simulink model "llm_inferencing_control"  (R2025b)
settings: Solver=FixedStepDiscrete  StartTime=0.0  StopTime=300  FixedStep=perturbed.dt  RelTol=1e-3
undefined symbols (not defined in the file): perturbed
settings Model: Creator=hvasudevan  LastModifiedBy=hvasudevan

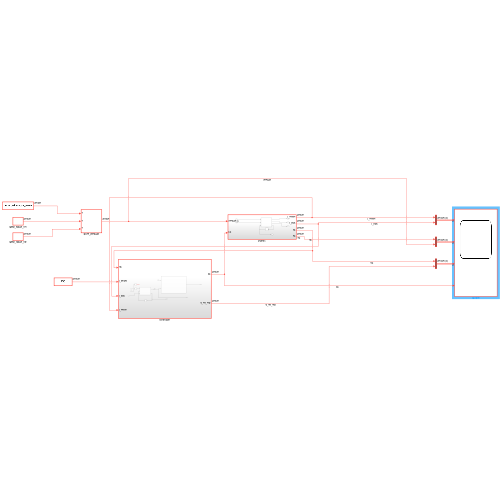
[thumbnail: Simulink's stored preview of the top-level diagram]
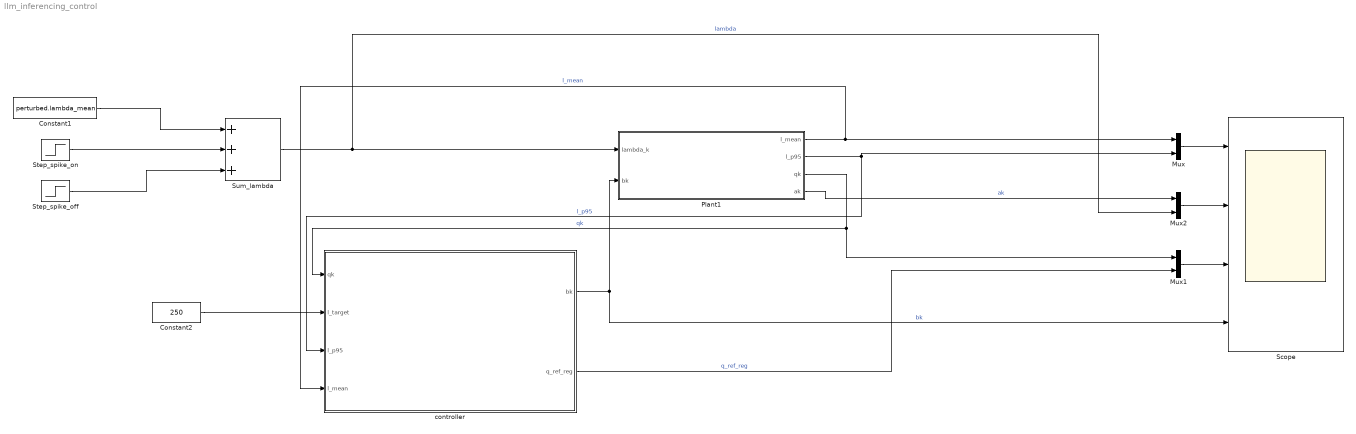
== system llm_inferencing_control ==
  Constant1 : Constant  Value=perturbed.lambda_mean  SampleTime=perturbed.dt
  Constant2 : Constant  Value=250  SampleTime=perturbed.dt
  Mux : Mux  Inputs=2
  Mux1 : Mux  Inputs=2
  Mux2 : Mux  Inputs=2
  Plant1 : Subsystem
  Scope : Scope  NumInputPorts=4
      settings: ActiveDisplayYMinimum=3.7725538298405183  ActiveDisplayYMaximum=466.04701553143548
  Step_spike_off : Step  Time=200  After=-perturbed.lambda_mean*1.5  SampleTime=perturbed.dt
  Step_spike_on : Step  Time=100  After=perturbed.lambda_mean*1.5  SampleTime=perturbed.dt
  Sum_lambda : Sum  Inputs=+++
  controller : Subsystem
  wires:
  Step_spike_off/1 -> Sum_lambda/3
  Plant1/3(qk) -> controller/1(qk), Mux1/1  "qk"
  Plant1/2(l_p95) -> Mux/2, controller/3(l_p95)  "l_p95"
  Plant1/1(l_mean) -> controller/4(l_mean), Mux/1  "l_mean"
  Step_spike_on/1 -> Sum_lambda/2
  Constant1/1 -> Sum_lambda/1
  Sum_lambda/1 -> Plant1/1(lambda_k), Mux2/2  "lambda"
  controller/1(bk) -> Scope/4, Plant1/2(bk)  "bk"
  Constant2/1 -> controller/2(l_target)
  Mux/1 -> Scope/1
  controller/2(q_ref_reg) -> Mux1/2  "q_ref_reg"
  Mux1/1 -> Scope/3
  Plant1/4(ak) -> Mux2/1  "ak"
  Mux2/1 -> Scope/2

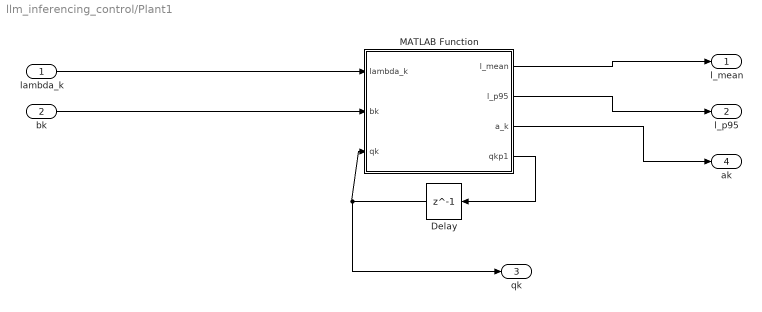
== system llm_inferencing_control/Plant1 ==
  lambda_k : Inport
  bk : Inport  Port=2
  Delay : Delay  DelayLength=1  InitialCondition=perturbed.q0  InputProcessing=Columns as channels (frame based)
  MATLAB Function : MATLAB Function  TreatAsAtomicUnit=on
  l_mean : Outport
  l_p95 : Outport  Port=2
  qk : Outport  Port=3
  ak : Outport  Port=4
  wires:
  MATLAB Function/2(l_p95) -> l_p95/1
  Delay/1 -> qk/1, MATLAB Function/3(qk)
  bk/1 -> MATLAB Function/2(bk)
  MATLAB Function/4(qkp1) -> Delay/1
  lambda_k/1 -> MATLAB Function/1(lambda_k)
  MATLAB Function/3(a_k) -> ak/1
  MATLAB Function/1(l_mean) -> l_mean/1

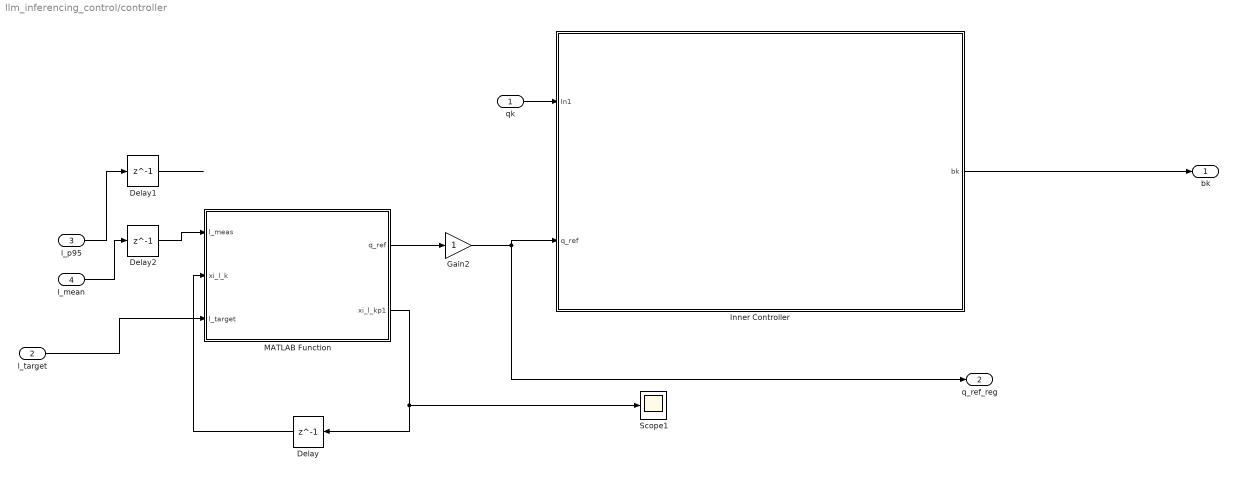
== system llm_inferencing_control/controller ==
  qk : Inport
  l_target : Inport  Port=2
  l_p95 : Inport  Port=3
  l_mean : Inport  Port=4
  Delay : Delay  DelayLength=1  InitialCondition=0  InputProcessing=Columns as channels (frame based)
  Delay1 : Delay  DelayLength=1  InitialCondition=50  InputProcessing=Columns as channels (frame based)
  Delay2 : Delay  DelayLength=1  InitialCondition=50  InputProcessing=Columns as channels (frame based)
  Gain2 : Gain
  Inner Controller : Subsystem
  MATLAB Function : MATLAB Function  TreatAsAtomicUnit=on
  Scope1 : Scope
      settings: ActiveDisplayYMinimum=-1  ActiveDisplayYMaximum=1  DataLoggingVariableName=ScopeData2
  bk : Outport
  q_ref_reg : Outport  Port=2
  wires:
  qk/1 -> Inner Controller/1(In1)
  MATLAB Function/2(xi_l_kp1) -> Scope1/1, Delay/1
  Delay/1 -> MATLAB Function/2(xi_l_k)
  Inner Controller/1(bk) -> bk/1
  Gain2/1 -> q_ref_reg/1, Inner Controller/2(q_ref)
  MATLAB Function/1(q_ref) -> Gain2/1
  l_mean/1 -> Delay2/1
  l_target/1 -> MATLAB Function/3(l_target)
  l_p95/1 -> Delay1/1
  Delay1/1 -> ?
  Delay2/1 -> MATLAB Function/1(l_meas)

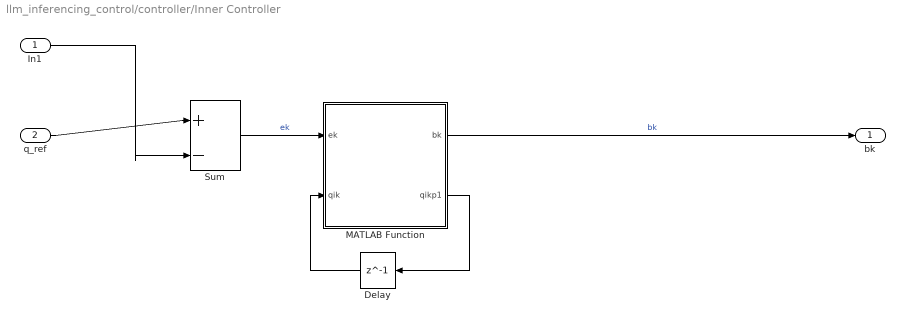
== system llm_inferencing_control/controller/Inner Controller ==
  In1 : Inport
  q_ref : Inport  Port=2
  Delay : Delay  DelayLength=1  InitialCondition=0  InputProcessing=Columns as channels (frame based)
  MATLAB Function : MATLAB Function  TreatAsAtomicUnit=on
  Sum : Sum  Inputs=|+-
  bk : Outport
  wires:
  MATLAB Function/2(qikp1) -> Delay/1
  q_ref/1 -> Sum/1
  In1/1 -> Sum/2
  MATLAB Function/1(bk) -> bk/1  "bk"
  Delay/1 -> MATLAB Function/2(qik)
  Sum/1 -> MATLAB Function/1(ek)  "ek"

== matlab function llm_inferencing_control/controller/Inner Controller/MATLAB Function ==
  data: ek input; qik input; bk output; controller parameter; qikp1 output
function [bk, qikp1] = inner_controller(ek, qik, controller)
q_max = controller.inner_c.q_max;
B0    = controller.inner_c.B0;
k_aug = controller.inner_c.K_aug;

% Saturate error and integrator state to [-q_max, q_max]
ek_sat  = min(max(ek,  -q_max), q_max);
qik_sat = min(max(qik, -q_max), q_max);

% Integrator update (Franklin 8.5.1: xi[k+1] = xi[k] + e[k])
qikp1 = qik_sat + ek_sat;

% Control law: B = B0 + K_aug * [ek; xi_k]
ek_vec = [ek_sat; qik_sat];
bk     = B0 + k_aug * ek_vec;

if(bk <= 1)
    bk = 1;
end

== matlab function llm_inferencing_control/controller/MATLAB Function ==
  data: l_meas input; q_ref output; xi_l_k input; l_target input; xi_l_kp1 output; controller parameter
function [q_ref, xi_l_kp1] = outer_controller(l_meas, xi_l_k, l_target, controller)
%OUTER_CONTROLLER Outer-loop latency controller with conditional anti-windup.
%
%   Inputs
%     l_meas    measured latency (mean or surrogate p95) [ms]
%     xi_l_k    current outer-loop integrator state
%     l_target  latency target [ms]
%     controller.outer_c  outer-controller parameter struct
%
%   Outputs
%     q_ref     commanded queue reference
%     xi_l_kp1  updated outer-loop integrator state
%
%   Control law:
%     e_l[k]        = l_target - l_meas[k]
%     xi_l[k+1]     = xi_l[k] + e_l[k]     (unless frozen by anti-windup)
%     Dq_ref[k]     = K_il * xi_l[k]
%     q_ref[k]      = q0 + Dq_ref[k]
%
%   Important lower-bound policy:
%     q_ref is NOT allowed to go to zero. In this setup, driving q_ref to 0
%     can effectively stall the inner loop / service action and make recovery
%     poor. Therefore the commanded queue reference is clamped to:
%
%       q_ref in [q_ref_min, q_max],   with q_ref_min = 1
%
%   Anti-windup logic:
%     - If q_ref is saturated at the lower limit and e_l would drive it
%       further downward, freeze the integrator.
%     - If q_ref is saturated at the upper limit and e_l would drive it
%       further upward, freeze the integrator.
%     - Otherwise integrate normally.
%
%   Since K_il > 0:
%     * more positive xi_l  -> larger q_ref
%     * more negative xi_l  -> smaller q_ref

q0       = controller.outer_c.q0;
q_max    = controller.outer_c.q_max;
K_il     = controller.outer_c.K_il;
xi_l_max = controller.outer_c.xi_l_max;
xi_l_min = controller.outer_c.xi_l_min;

% Minimum allowed outer-loop queue reference.
% Using 1 instead of 0 avoids complete shutdown of queue demand.
q_ref_min = 1;

% Latency error
e_l = l_target - l_meas;

% Clamp integrator to absolute safe bounds first
xi_l_sat = min(max(xi_l_k, xi_l_min), xi_l_max);

% Unsaturated control from current integrator state
dq_ref_unsat = K_il * xi_l_sat;
q_ref_unsat  = q0 + dq_ref_unsat;

% Saturated control actually applied
q_ref = min(max(q_ref_unsat, q_ref_min), q_max);

% Conditional integration anti-windup
% Freeze only when the actuator is at a limit AND the current error would
% push it further into that same limit.
freeze_low  = (q_ref <= q_ref_min) && (e_l < 0);
freeze_high = (q_ref >= q_max)     && (e_l > 0);

if freeze_low || freeze_high
    xi_l_kp1 = xi_l_sat;   % freeze integrator at the boundary
else
    xi_l_kp1 = xi_l_sat + e_l;
    xi_l_kp1 = min(max(xi_l_kp1, xi_l_min), xi_l_max);
end

end

== matlab function llm_inferencing_control/Plant1/MATLAB Function ==
  data: lambda_k input; bk input; l_mean output; qk input; l_p95 output; a_k output; qkp1 output; perturbed parameter
function [l_mean, l_p95, a_k, qkp1] = fcn(lambda_k, bk, qk, perturbed)
%% STATISTICAL PLANT - Chapter 2
%% Replaces deterministic arrivals and closed-form p95 with:
%%   - True Poisson arrivals: a[k] ~ Poisson(lambda_k)
%%   - Per-tick latency sample with additive noise
%%   - Empirical rolling p95 over a 60-sample window
%%
%% Everything else (queue equation, latency formula, parameters)
%% is identical to Chapter 1.

persistent L_buf buf_idx buf_full
N = 20;
if isempty(L_buf)
    %% Warm-start buffer at target so outer loop sees zero error at t=0.
    %% Without this the cold buffer reads L_p95~0 and winds the integrator.
    L_buf    = perturbed.L_p95_target * ones(1, N);
    buf_idx  = 0;
    buf_full = true;
end

alpha = perturbed.alpha;
gam   = perturbed.gamma;
beta  = perturbed.beta;
delta = perturbed.delta;

%% True Poisson arrivals (not Gaussian approx — avoids fat-tail spikes)
a_k = poissrnd(max(0, lambda_k));

%% Queue state equation — identical to Chapter 1
qkp1 = max(0, qk + a_k - bk);

%% Latency sample this tick
bk_safe = max(1, bk);
l_det   = alpha*bk + gam*bk^2 + beta*qk;
l_samp  = l_det + (delta / sqrt(bk_safe)) * randn();

%% Update circular buffer
buf_idx = mod(buf_idx, N) + 1;
L_buf(buf_idx) = l_samp;

%% Rolling statistics
if buf_full
    data = L_buf;
else
    data = L_buf(1 : buf_idx);
end

l_mean = mean(data);
sorted = sort(data);
idx95  = max(1, ceil(0.95 * length(sorted)));
l_p95  = sorted(idx95);

end
